simulink model "PID_Angle"  (Simulink 7.9)
settings: Solver=ode45  StartTime=0.0  StopTime=10  RelTol=1e-3
undefined symbols (not defined in the file): A, Kd, v
libraries: simulink x1
settings Model: Creator=dave  LastModifiedBy=dave

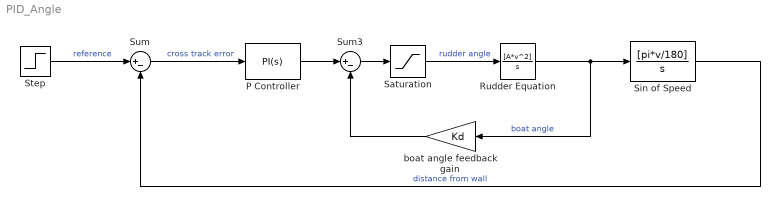
== system PID_Angle ==
  P Controller : simulink/Continuous/PID Controller  Controller=PI  TimeDomain=Continuous-time  SampleTime=1  IntegratorMethod=Forward Euler  FilterMethod=Forward Euler  Form=Parallel  P=2.6  I=0.3  D=0  N=7.02962681019428  InitialConditionSource=internal  InitialConditionForIntegrator=0  InitialConditionForFilter=0  ExternalReset=none  LimitOutput=off  UpperSaturationLimit=inf  LowerSaturationLimit=-inf  LinearizeAsGain=off  AntiWindupMode=none  Kb=1  TrackingMode=off  Kt=1  PParamMin=[]  PParamMax=[]  IParamMin=[]  IParamMax=[]  DParamMin=[]  DParamMax=[]  NParamMin=[]  NParamMax=[]  KbParamMin=[]  KbParamMax=[]  KtParamMin=[]  KtParamMax=[]  POutMin=[]  POutMax=[]  IOutMin=[]  IOutMax=[]  DOutMin=[]  DOutMax=[]  NOutMin=[]  NOutMax=[]  KbOutMin=[]  KbOutMax=[]  KtOutMin=[]  KtOutMax=[]  IntegratorOutMin=[]  IntegratorOutMax=[]  FilterOutMin=[]  FilterOutMax=[]  SumOutMin=[]  SumOutMax=[]  SumI1OutMin=[]  SumI1OutMax=[]  SumI2OutMin=[]  SumI2OutMax=[]  SumI3OutMin=[]  SumI3OutMax=[]  SumDOutMin=[]  SumDOutMax=[]  SaturationOutMin=[]  SaturationOutMax=[]  IntegratorContinuousStateAttributes=''  IntegratorStateMustResolveToSignalObject=off  IntegratorRTWStateStorageClass=Auto  FilterContinuousStateAttributes=''  FilterStateMustResolveToSignalObject=off  FilterRTWStateStorageClass=Auto
  Rudder Equation : TransferFcn  Numerator=[A*v^2]  Denominator=[1 0]
  Saturation : Saturate  UpperLimit=25  LowerLimit=-25
  Sin of Speed : TransferFcn  Numerator=[pi*v/180]  Denominator=[1 0]
  Step : Step  SampleTime=0
  Sum : Sum  Inputs=|+-
  Sum3 : Sum  Inputs=|+-
  boat angle feedback gain : Gain  Gain=Kd
  wires:
  Sum/1 -> P Controller/1  "cross track error"
  Step/1 -> Sum/1  "reference"
  Saturation/1 -> Rudder Equation/1  "rudder angle"
  P Controller/1 -> Sum3/1
  Sum3/1 -> Saturation/1
  boat angle feedback gain/1 -> Sum3/2
  Rudder Equation/1 -> boat angle feedback gain/1, Sin of Speed/1  "boat angle"
  Sin of Speed/1 -> Sum/2  "distance from wall"
